simulink model "coilsim_slx"  (R2022a)
settings: Solver=VariableStepAuto  StartTime=0.0  StopTime=tmax  FixedStep=sampletime  RelTol=1e-3
values from neighbouring files (symbols this model uses):
  Cc = eye(tok.nc, tok.nc+tok.nv)    [cc_analysis.m]    (also in run_coilsim.m = eye(size(K,2), size(G,1)); vac_step_response.m)
  G = ss(A,B,eye(size(A)), 0)    [cc_analysis.m]    (also in close_vs_loops.m = reduce(G, opt.model_order); optimize_vec.m = struct2vec(C, fds); run_coilsim.m = ss(G); test_vs_optimization2.m = {})
  K = ss(K)    [cc_analysis.m]    (also in nstxu_coilcontrol_lqi.m = Kp + Ki/s; nstxu_coilcontrol_lqr.m = K(:,1:tok.nc); nstxu_coilcontrol_pid.m = Kp + Ki/s + Kd*s/(tauroll*s + 1); run_coilsim.m)
  ref = zeros(tok.nc,1)    [cc_analysis.m]    (also in shape_cinv_controlsim.m = struct2vec(targ, y_fds); vac_step_response.m)
  vmax = circ.vmax    [cc_analysis.m]    (also in vac_step_response.m)
  vmin = circ.vmin    [cc_analysis.m]    (also in vac_step_response.m)
settings Model: Creator=jwai  LastModifiedBy=jwai

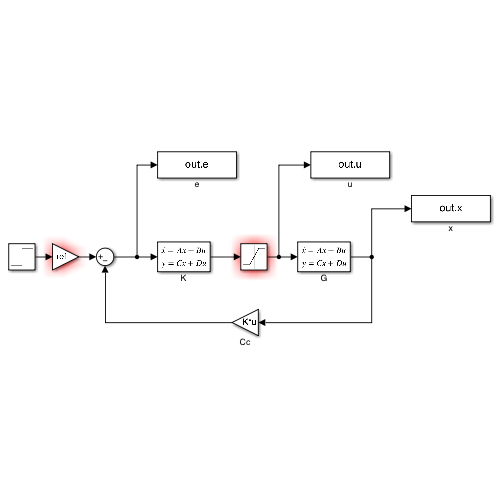
[thumbnail: Simulink's stored preview of the top-level diagram]
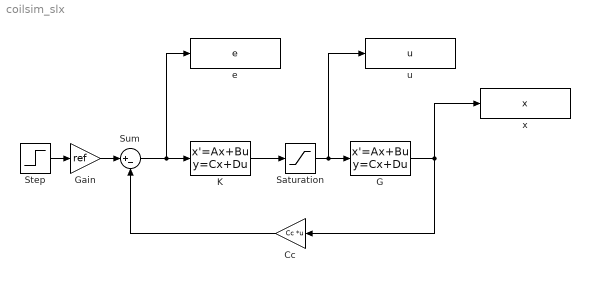
== system coilsim_slx ==
  Cc : Gain  Gain=Cc  Multiplication=Matrix(K*u)
  G : StateSpace  A=G.A  B=G.B  C=G.C  D=G.D  InitialCondition=0
  Gain : Gain  Gain=ref
  K : StateSpace  A=K.A  B=K.B  C=K.C  D=K.D  InitialCondition=0
  Saturation : Saturate  UpperLimit=vmax  LowerLimit=vmin
  Step : Step  Time=0  SampleTime=0
  Sum : Sum  Inputs=|+-
  e : ToWorkspace  VariableName=e  SaveFormat=Timeseries  SampleTime=-1
  u : ToWorkspace  VariableName=u  SaveFormat=Timeseries  SampleTime=-1
  x : ToWorkspace  VariableName=x  SaveFormat=Timeseries  SampleTime=-1
  wires:
  Step/1 -> Gain/1
  K/1 -> Saturation/1
  Saturation/1 -> u/1, G/1
  Gain/1 -> Sum/1
  G/1 -> Cc/1, x/1
  Sum/1 -> e/1, K/1
  Cc/1 -> Sum/2
